simulink model "VCMGCM1962020b_v2"  (R2020b)
settings: Solver=FixedStepDiscrete  StartTime=0.0  StopTime=10.0  FixedStep=0.005  RelTol=1e-3  EnableMultiTasking=on
PreLoadFcn:
  | try, model_open; catch, disp('Error occurred while executing model pre-load callback: model_open.m'); disp('Please assure that the MATLAB working directory is set to the model directory before opening.'); end
InitFcn:
  | try, model_open; catch, end
undefined symbols (not defined in the file): Bridge, GCM, H, raptor_get_param_eval, raptor_get_safe_string, raptor_xcp_function
libraries: Blocks_lib x1165, Raptor_lib x665, simulink x62, VCM_lib x5
(part 8 of 23)

== system VCMGCM1962020b_v2/Fgnd/Actuators/CAN/Other/MPDM ==
  Data : Inport
  Ground : Ground
  Header : Blocks_lib/Header  width=Portrait  addtext=''
  MsgName : Subsystem
      mask help:
      | Example of how to set up a CAN message transmit.
      | 1. Copy this block into the main model.
      | 2. Disable/break library link.
      | 3. Underneath, set up CAN Tx Message block.
      | 4. For each field, connect a CANTxField block from the CAN block to the bus creator; adjust parameters as necessary.
      mask init:
      | [msgnam, msgbus] = CANBlockInit('Tx');
      mask Display: disp(['CAN Tx: Message\n' msgnam '\n' msgbus]);
  Act : Outport  VectorParamsAs1DForOutWhenUnconnected=off
  wires:
  Data/1 -> MsgName/1(Data)
  Ground/1 -> Act/1  "MPDM"

== system VCMGCM1962020b_v2/Fgnd/Actuators/CAN/Other/Power Steering Pump Inverter ==
  Data : Inport
  Ground : Ground
  Header : Blocks_lib/Header  width=Portrait  addtext=''
  MsgName : Subsystem
      mask help:
      | Example of how to set up a CAN message transmit.
      | 1. Copy this block into the main model.
      | 2. Disable/break library link.
      | 3. Underneath, set up CAN Tx Message block.
      | 4. For each field, connect a CANTxField block from the CAN block to the bus creator; adjust parameters as necessary.
      mask init:
      | [msgnam, msgbus] = CANBlockInit('Tx');
      mask Display: disp(['CAN Tx: Message\n' msgnam '\n' msgbus]);
  PSPInvtrHC1_Demands : Subsystem
      mask help:
      | Example of how to set up a CAN message transmit.
      | 1. Copy this block into the main model.
      | 2. Disable/break library link.
      | 3. Underneath, set up CAN Tx Message block.
      | 4. For each field, connect a CANTxField block from the CAN block to the bus creator; adjust parameters as necessary.
      mask init:
      | [msgnam, msgbus] = CANBlockInit('Tx');
      mask Display: disp(['CAN Tx: Message\n' msgnam '\n' msgbus]);
  PSPInvtrHC3_Battery_Demands : Subsystem
      mask help:
      | Example of how to set up a CAN message transmit.
      | 1. Copy this block into the main model.
      | 2. Disable/break library link.
      | 3. Underneath, set up CAN Tx Message block.
      | 4. For each field, connect a CANTxField block from the CAN block to the bus creator; adjust parameters as necessary.
      mask init:
      | [msgnam, msgbus] = CANBlockInit('Tx');
      mask Display: disp(['CAN Tx: Message\n' msgnam '\n' msgbus]);
  Act : Outport  VectorParamsAs1DForOutWhenUnconnected=off
  wires:
  Ground/1 -> Act/1  "PSPInvtr"
  Data/1 -> PSPInvtrHC1_Demands/1(Data), MsgName/1(Data), PSPInvtrHC3_Battery_Demands/1(Data)

== system VCMGCM1962020b_v2/Fgnd/Actuators/FMWS/MCU_130h/FMWS Enbl ==
  note: Vehicle is moving or ready to move
  note: Vehicle is moving while in neutral
  note: First two conditions being true would mean vehicle is in neutral
  In1 : Inport
  AND1 : Logic  Inputs=3  AllPortsSameDT=off  OutDataTypeStr=boolean
  Bus Selector : BusSelector  OutputSignals=Control.Mode.StartStop.RunMode [Bool],VirtualSensors.Driver.Drv [Bool],VirtualSensors.Driver.Rev [Bool],VirtualSensors.Spd.VehSpd [kph]
  Compare To Zero : simulink/Logic and Bit Operations/Compare To Zero  relop=>  OutDataTypeStr=boolean
  NOT : Logic  Operator=NOT  IconShape=distinctive  AllPortsSameDT=off  OutDataTypeStr=boolean
  NOT1 : Logic  Operator=NOT  IconShape=distinctive  AllPortsSameDT=off  OutDataTypeStr=boolean
  OR : Logic  Operator=OR  AllPortsSameDT=off  OutDataTypeStr=boolean
  raptor_measurement : Raptor_lib/Data Storage/raptor_measurement  paramName='FMWS_Enbl'  nameSource=Parameter  calDispType=Number  calEnum={'False', 'True'}  calGain=1.0  calOffset=0.0  calMax=inf  calMin=-inf  calFormat='-1'  calUnit='Enable condition met for FMWS'  calHelp='Enable condition met for FMWS'  calAccess=1  calFunction=raptor_xcp_function(gcb)  calVisible=on
      settings: SourceProductName=Raptor
  raptor_override : Raptor_lib/Data Storage/raptor_override  paramName='FMWS_Enbl'  nameSource=Parameter  measurement=None  calDispType=Number  calEnum={'False', 'True'}  calGain=1.0  calOffset=0.0  calMax=inf  calMin=-inf  calFormat='-1'  calUnit='Enable condition met for FMWS'  calHelp='Enable condition met for FMWS'  calAccess=1  calFunction="[raptor_xcp_function(gcb) '|'  'Override']"
      settings: SourceProductName=Raptor
  Out1 : Outport
  wires:
  NOT1/1 -> AND1/2
  Bus Selector/2 -> NOT/1  "<Drv [Bool]>"
  Bus Selector/3 -> NOT1/1  "<Rev [Bool]>"
  AND1/1 -> OR/2
  In1/1 -> Bus Selector/1
  Bus Selector/1 -> OR/1  "<RunMode [Bool]>"
  NOT/1 -> AND1/1
  Bus Selector/4 -> Compare To Zero/1  "<VehSpd [kph]>"
  Compare To Zero/1 -> AND1/3
  raptor_override/1 -> raptor_measurement/1, Out1/1
  OR/1 -> raptor_override/1

== system VCMGCM1962020b_v2/Fgnd/Actuators/FMWS/MCU_130h/MsgTx ==
  Data : Inport
  Enable : EnablePort
  Bus Selector : BusSelector  OutputSignals=Control.Other.Other.FMWS_StateGear [enum]
  CANTxField1 : Blocks_lib/CANTxField  custom=off  custom_nam='---'  custom_units='---'
  Header : Blocks_lib/Header  width=Landscape  addtext=''
  raptor_can_txmsg : Raptor_lib/CAN/raptor_can_txmsg  canDefinition=struct('dbcFile', 'FMWS.dbc','message', 'MCU_130h','comment', '','signals', {{'MCU_MotActuSpd','GearPos'}},'enabled', [ 0 1;],'scaled', [ 1 1;],'canBus', 'bus','messageID', [ 304;],'idMask', [ 536870911;],'payloadMask', [],'payloadValue', [],'period', [ 100;],'mailbox', '','queueSize', [ 1;],'label', [ 1;],'ver', [ 2;],'showID', [ 0;],'showRaw', [ 0;],'fill', [ 0;],'editID', [ 0;],'signalOrder', [ 3;],'signalAscDes', [ 1;])  canBus=bus  queueSize=1  payloadMask=[]  payloadValue=[]  period=100  showID=0  label=1  idMask=hex2dec('1FFFFFFF')  fill=0  id=304  showRaw=0  signalOrder=3  signalInfo={{struct('Name', 'MCU_MotActuSpd','Startbit', [ 0;],'SignalSize', [ 16;],'ByteOrder', 'LittleEndian','ValueType', 'UNSIGNED','Class', 'uint16','Signed', [ 0;],'Factor', [ 1;],'Offset', [ -32000;],'Min', [ -32000;],'Max', [ 32000;],'Units', 'Rpm','Comment', 'Motor actual speed','StartBit', [ 16;]),struct('Name', 'GearPos','Startbit', [ 0;],'SignalSize', [ 8;],'ByteOrder', 'LittleEndian','ValueType', 'UNSIGNED','Class', 'uint8','Signed', [ 0;],'Factor', [ 1;],'Offset', [ 0;],'Min', [ 0;],'Max', [ 0;],'Units', '','Comment', '','StartBit', [ 48;])}}
      settings: SourceProductName=Raptor
  wires:
  Data/1 -> Bus Selector/1
  CANTxField1/1 -> raptor_can_txmsg/1  "GearPos"
  Bus Selector/1 -> CANTxField1/1  "<FMWS_StateGear [enum]>"

== system VCMGCM1962020b_v2/Fgnd/Actuators/FMWS/MCU_131h/MsgTx ==
  Data : Inport
  Enable : EnablePort
  Bus Selector : BusSelector  OutputSignals=VirtualSensors.Spd.VehSpd [kph]
  CANTxField : Blocks_lib/CANTxField  custom=on  custom_nam=[nam '---']  custom_units='---'
  Header : Blocks_lib/Header  width=Landscape  addtext=''
  raptor_can_txmsg : Raptor_lib/CAN/raptor_can_txmsg  canDefinition=struct('dbcFile', 'FMWS.dbc','message', 'MCU_131h','comment', '','signals', {{'VehicleSpeed'}},'enabled', [ 1;],'scaled', [ 1;],'canBus', 'bus','messageID', [ 305;],'idMask', [ 536870911;],'payloadMask', [],'payloadValue', [],'period', [ 100;],'queueSize', [ 1;],'label', [ 1;],'ver', [ 2;],'showID', [ 0;],'showRaw', [ 0;],'showRawMsg', [ 0;],'useStartVals', [ 0;],'useSimFunc', [ 0;],'sim_func_name', '''''','fill', [ 0;],'editID', [ 0;],'signalOrder', [ 3;],'signalAscDes', [ 1;],'msgLength', [ 8;])  canBus=bus  queueSize=1  payloadMask=[]  payloadValue=[]  period=100  showID=0  label=1  idMask=hex2dec('1FFFFFFF')  fill=0  id=305  showRaw=0  signalOrder=3  signalInfo={{struct('Name', 'VehicleSpeed','Startbit', [ 0;],'SignalSize', [ 16;],'ByteOrder', 'LittleEndian','ValueType', 'SIGNED','Class', 'int16','Signed', [ 1;],'Factor', [ 0.0625;],'Offset', [ 0;],'Min', [ -100;],'Max', [ 100;],'Units', 'Km/hr','Comment', 'Speed','StartBit', [ 0;])}}
      settings: SourceProductName=Raptor
  wires:
  Bus Selector/1 -> CANTxField/1  "<VehSpd [kph]>"
  Data/1 -> Bus Selector/1
  CANTxField/1 -> raptor_can_txmsg/1  "VehicleSpeed"

== system VCMGCM1962020b_v2/Fgnd/Actuators/FMWS_J1939/CCVS/MsgTx ==
  Data : Inport
  Enable : EnablePort
  Bus Selector : BusSelector  OutputSignals=VirtualSensors.Spd.VehSpd [kph],VirtualSensors.Driver.Prk [Bool]
  CANTxField1 : Blocks_lib/CANTxField  custom=off  custom_nam='---'  custom_units='---'
  CANTxField2 : Blocks_lib/CANTxField  custom=off  custom_nam='---'  custom_units='---'
  Header : Blocks_lib/Header  width=Landscape  addtext=''
  raptor_can_txmsg : Raptor_lib/CAN/raptor_can_txmsg  canDefinition=struct('dbcFile', 'ECCO_EVAS.dbc','message', 'CCVS','comment', '','signals', {{'EngShutdownOverrideSwitch','EngTestModeSwitch','EngIdleDecrementSwitch','EngIdleIncrementSwitch','CruiseCtrlStates','PTOGovernorState','CruiseCtrlSetSpeed','CruiseCtrlAccelerateSwitch','CruiseCtrlResumeSwitch','CruiseCtrlCoastSwitch','CruiseCtrlSetSwitch','ClutchSwitch','BrakeSwitch','CruiseCtrlEnableSwitch','CruiseCtrlActive','WheelBasedVehicleSpeed','ParkBrakeReleaseInhibitRq','CruiseCtrlPauseSwitch','ParkingBrakeSwitch','TwoSpeedAxleSwitch'}},'enabled', [ 0 0 0 0 0 0 0 0 0 0 0 0 0 0 0 1 0 0 1 0;],'scaled', [ 1 1 1 1 1 1 1 1 1 1 1 1 1 1 1 1 1 1 1 1;],'canBus', 'bus','messageID', [ 419361024;],'idMask', [ 536870911;],'payloadMask', [],'payloadValue', [],'period', [ 100;],'mailbox', '','queueSize', [ 1;],'label', [ 1;],'ver', [ 2;],'showID', [ 0;],'showRaw', [ 0;],'fill', [ 0;],'editID', [ 0;],'signalOrder', [ 3;],'signalAscDes', [ 1;])  canBus=bus  queueSize=1  payloadMask=[]  payloadValue=[]  period=100  showID=0  label=1  idMask=hex2dec('1FFFFFFF')  fill=0  id=419361024  showRaw=0  signalOrder=3  signalInfo={{struct('Name', 'EngShutdownOverrideSwitch','Startbit', [ 0;],'SignalSize', [ 2;],'ByteOrder', 'LittleEndian','ValueType', 'UNSIGNED','Class', 'uint8','Signed', [ 0;],'Factor', [ 1;],'Offset', [ 0;],'Min', [ 0;],'Max', [ 3;],'Units', '','Comment', '','StartBit', [ 62;]),struct('Name', 'EngTestModeSwitch','Startbit', [ 0;],'SignalSize', [ 2;],'ByteOrder', 'LittleEndian','ValueType', 'UNSIGNED','Class', 'uint8','Signed', [ 0;],'Factor', [ 1;],'Offset', [ 0;],'Min', [ 0;],'Max', [ 3;],'Units', '','Comment', '','StartBit', [ 60;]),struct('Name', 'EngIdleDecrementSwitch','Startbit', [ 0;],'SignalSize', [ 2;],'ByteOrder', 'LittleEndian','ValueType', 'UNSIGNED','Class', 'uint8','Signed', [ 0;],'Factor', [ 1;],'Offset', [ 0;],'Min', [ 0;],'Max', [ 3;],'Units', '','Comment', '','StartBit', [ 58;]),struct('Name', 'EngIdleIncrementSwitch','Startbit', [ 0;],'SignalSize', [ 2;],'ByteOrder', 'LittleEndian','ValueType', 'UNSIGNED','Class', 'uint8','Signed', [ 0;],'Factor', [ 1;],'Offset', [ 0;],'Min', [ 0;],'Max', [ 3;],'Units', '','Comment', '','StartBit', [ 56;]),struct('Name', 'CruiseCtrlStates','Startbit', [ 0;],'SignalSize', [ 3;],'ByteOrder', 'LittleEndian','ValueType', 'UNSIGNED','Class', 'uint8','Signed', [ 0;],'Factor', [ 1;],'Offset', [ 0;],'Min', [ 0;],'Max', [ 7;],'Units', '','Comment', '','StartBit', [ 53;]),struct('Name', 'PTOGovernorState','Startbit', [ 0;],'SignalSize', [ 5;],'ByteOrder', 'LittleEndian','ValueType', 'UNSIGNED','Class', 'uint8','Signed', [ 0;],'Factor', [ 1;],'Offset', [ 0;],'Min', [ 0;],'Max', [ 31;],'Units', '','Comment', '','StartBit', [ 48;]),struct('Name', 'CruiseCtrlSetSpeed','Startbit', [ 0;],'SignalSize', [ 8;],'ByteOrder', 'LittleEndian','ValueType', 'UNSIGNED','Class', 'uint8','Signed', [ 0;],'Factor', [ 1;],'Offset', [ 0;],'Min', [ 0;],'Max', [ 250;],'Units', 'km/h','Comment', '','StartBit', [ 40;]),struct('Name', 'CruiseCtrlAccelerateSwitch','Startbit', [ 0;],'SignalSize', [ 2;],'ByteOrder', 'LittleEndian','ValueType', 'UNSIGNED','Class', 'uint8','Signed', [ 0;],'Factor', [ 1;],'Offset', [ 0;],'Min', [ 0;],'Max', [ 3;],'Units', '','Comment', '','StartBit', [ 38;]),struct('Name', 'CruiseCtrlResumeSwitch','Startbit', [ 0;],'SignalSize', [ 2;],'ByteOrder', 'LittleEndian','ValueType', 'UNSIGNED','Class', 'uint8','Signed', [ 0;],'Factor', [ 1;],'Offset', [ 0;],'Min', [ 0;],'Max', [ 3;],'Units', '','Comment', '','StartBit', [ 36;]),struct('Name', 'CruiseCtrlCoastSwitch','Startbit', [ 0;],'SignalSize', [ 2;],'ByteOrder', 'LittleEndian','ValueType', 'UNSIGNED','Class', 'uint8','Signed', [ 0;],'Factor', [ 1;],'Offset', [ 0;],'Min', [ 0;],'Max', [ 3;],'Units', '','Comment', '','StartBit', [ 34;]),struct('Name', 'CruiseCtrlSetSwitch','Startbit', [ 0;],'SignalSize', [ 2;],'ByteOrder', 'LittleEndian','ValueType', 'UNSIGNED','Class', 'uint8','Signed', [ 0;],'Factor', [ 1;],'Offset', [ 0;],'Min', [ 0;],'Max', [ 3;],'Units', '','Comment', '','StartBit', [ 32;]),struct('Name', 'ClutchSwitch','Startbit', [ 0;],'SignalSize', [ 2;],'ByteOrder', 'LittleEndian','ValueType', 'UNSIGNED','Class', 'uint8','Signed', [ 0;],'Factor', [ 1;],'Offset', [ 0;],'Min', [ 0;],'Max', [ 3;],'Units', '','Comment', '','StartBit', [ 30;]),struct('Name', 'BrakeSwitch','Startbit', [ 0;],'SignalSize', [ 2;],'ByteOrder', 'LittleEndian','ValueType', 'UNSIGNED','Class', 'uint8','Signed', [ 0;],'Factor', [ 1;],'Offset', [ 0;],'Min', [ 0;],'Max', [ 3;],'Units', '','Comment', '','StartBit', [ 28;]),struct('Name', 'CruiseCtrlEnableSwitch','Startbit', [ 0;],'SignalSize', [ 2;],'ByteOrder', 'LittleEndian','ValueType', 'UNSIGNED','Class', 'uint8','Signed', [ 0;],'Factor', [ 1;],'Offset', [ 0;],'Min', [ 0;],'Max', [ 3;],'Units', '','Comment', '','StartBit', [ 26;]),struct('Name', 'CruiseCtrlActive','Startbit', [ 0;],'SignalSize', [ 2;],'ByteOrder', 'LittleEndian','ValueType', 'UNSIGNED','Class', 'uint8','Signed', [ 0;],'Factor', [ 1;],'Offset', [ 0;],'Min', [ 0;],'Max', [ 3;],'Units', '','Comment', '','StartBit', [ 24;]),struct('Name', 'WheelBasedVehicleSpeed','Startbit', [ 0;],'SignalSize', [ 16;],'ByteOrder', 'LittleEndian','ValueType', 'UNSIGNED','Class', 'uint16','Signed', [ 0;],'Factor', [ 0.0039062;],'Offset', [ 0;],'Min', [ 0;],'Max', [ 250.996;],'Units', 'km/h','Comment', '','StartBit', [ 8;]),struct('Name', 'ParkBrakeReleaseInhibitRq','Startbit', [ 0;],'SignalSize', [ 2;],'ByteOrder', 'LittleEndian','ValueType', 'UNSIGNED','Class', 'uint8','Signed', [ 0;],'Factor', [ 1;],'Offset', [ 0;],'Min', [ 0;],'Max', [ 3;],'Units', '','Comment', '','StartBit', [ 6;]),struct('Name', 'CruiseCtrlPauseSwitch','Startbit', [ 0;],'SignalSize', [ 2;],'ByteOrder', 'LittleEndian','ValueType', 'UNSIGNED','Class', 'uint8','Signed', [ 0;],'Factor', [ 1;],'Offset', [ 0;],'Min', [ 0;],'Max', [ 3;],'Units', '','Comment', '','StartBit', [ 4;]),struct('Name', 'ParkingBrakeSwitch','Startbit', [ 0;],'SignalSize', [ 2;],'ByteOrder', 'LittleEndian','ValueType', 'UNSIGNED','Class', 'uint8','Signed', [ 0;],'Factor', [ 1;],'Offset', [ 0;],'Min', [ 0;],'Max', [ 3;],'Units', '','Comment', '','StartBit', [ 2;]),struct('Name', 'TwoSpeedAxleSwitch','Startbit', [ 0;],'SignalSize', [ 2;],'ByteOrder', 'LittleEndian','ValueType', 'UNSIGNED','Class', 'uint8','Signed', [ 0;],'Factor', [ 1;],'Offset', [ 0;],'Min', [ 0;],'Max', [ 3;],'Units', '','Comment', '','StartBit', [ 0;])}}
      settings: SourceProductName=Raptor
  wires:
  CANTxField1/1 -> raptor_can_txmsg/1  "WheelBasedVehicleSpeed"
  Data/1 -> Bus Selector/1
  Bus Selector/2 -> CANTxField2/1  "<Prk [Bool]>"
  CANTxField2/1 -> raptor_can_txmsg/2  "ParkingBrakeSwitch"
  Bus Selector/1 -> CANTxField1/1  "<VehSpd [kph]>"

== system VCMGCM1962020b_v2/Fgnd/Actuators/FMWS_J1939/ETC2/MsgTx ==
  Data : Inport
  Enable : EnablePort
  Bus Selector : BusSelector  OutputSignals=VirtualSensors.Spd.VehSpd [kph]
  CANTxField : Blocks_lib/CANTxField  custom=on  custom_nam=[nam '---']  custom_units='---'
  Header : Blocks_lib/Header  width=Landscape  addtext=''
  raptor_can_txmsg : Raptor_lib/CAN/raptor_can_txmsg  canDefinition=struct('dbcFile', 'ECCO_EVAS.dbc','message', 'ETC2','comment', '','signals', {{'TransCurrentRange','TransRequestedRange','TransCurrentGear','TransActualGearRatio','TransSelectedGear'}},'enabled', [ 0 0 1 0 0;],'scaled', [ 1 1 1 1 1;],'canBus', 'bus','messageID', [ 418383104;],'idMask', [ 536870911;],'payloadMask', [],'payloadValue', [],'period', [ 100;],'mailbox', '','queueSize', [ 1;],'label', [ 1;],'ver', [ 2;],'showID', [ 0;],'showRaw', [ 0;],'fill', [ 0;],'editID', [ 0;],'signalOrder', [ 3;],'signalAscDes', [ 1;])  canBus=bus  queueSize=1  payloadMask=[]  payloadValue=[]  period=100  showID=0  label=1  idMask=hex2dec('1FFFFFFF')  fill=0  id=418383104  showRaw=0  signalOrder=3  signalInfo={{struct('Name', 'TransCurrentRange','Startbit', [ 0;],'SignalSize', [ 16;],'ByteOrder', 'LittleEndian','ValueType', 'UNSIGNED','Class', 'uint16','Signed', [ 0;],'Factor', [ 1;],'Offset', [ 0;],'Min', [ 0;],'Max', [ 255;],'Units', 'per byte','Comment', '','StartBit', [ 48;]),struct('Name', 'TransRequestedRange','Startbit', [ 0;],'SignalSize', [ 16;],'ByteOrder', 'LittleEndian','ValueType', 'UNSIGNED','Class', 'uint16','Signed', [ 0;],'Factor', [ 1;],'Offset', [ 0;],'Min', [ 0;],'Max', [ 255;],'Units', 'per byte','Comment', '','StartBit', [ 32;]),struct('Name', 'TransCurrentGear','Startbit', [ 0;],'SignalSize', [ 8;],'ByteOrder', 'LittleEndian','ValueType', 'UNSIGNED','Class', 'uint8','Signed', [ 0;],'Factor', [ 1;],'Offset', [ -125;],'Min', [ -125;],'Max', [ 125;],'Units', '','Comment', '','StartBit', [ 24;]),struct('Name', 'TransActualGearRatio','Startbit', [ 0;],'SignalSize', [ 16;],'ByteOrder', 'LittleEndian','ValueType', 'UNSIGNED','Class', 'uint16','Signed', [ 0;],'Factor', [ 0.001;],'Offset', [ 0;],'Min', [ 0;],'Max', [ 64.255;],'Units', '','Comment', '','StartBit', [ 8;]),struct('Name', 'TransSelectedGear','Startbit', [ 0;],'SignalSize', [ 8;],'ByteOrder', 'LittleEndian','ValueType', 'UNSIGNED','Class', 'uint8','Signed', [ 0;],'Factor', [ 1;],'Offset', [ -125;],'Min', [ -125;],'Max', [ 125;],'Units', '','Comment', '','StartBit', [ 0;])}}
      settings: SourceProductName=Raptor
  wires:
  CANTxField/1 -> raptor_can_txmsg/1  "TransCurrentGear"
  Data/1 -> Bus Selector/1
  Bus Selector/1 -> CANTxField/1  "<VehSpd [kph]>"

== system VCMGCM1962020b_v2/Fgnd/Control/Drive Inverter/Motor Torque Request/Current//Torque Split ==
  Data : Inport
  TrqReq : Inport  Port=2
  Bus Creator : BusCreator  Inputs=3
  Bus Selector : BusSelector  OutputSignals=DrvTrqReqFinal [Nm]
  Constant : Constant  Value=double(1)
  Constant1 : Constant  Value=double(1)
  Constant2 : Constant  Value=double(1)
  Header : Blocks_lib/Header  width=Portrait  addtext=''
  Inverter Current Limits : Subsystem
  Product : Product
  Product1 : Product
  Product2 : Product
  Split : Outport  VectorParamsAs1DForOutWhenUnconnected=off
  wires:
  Product/1 -> Bus Creator/1  "DrvInvtrMCLSplit [A]"
  Bus Creator/1 -> Split/1  "Split"
  Product1/1 -> Bus Creator/2  "DrvInvtrGCLSplit [A]"
  Product2/1 -> Bus Creator/3  "DrvMtrTrqReqSplit [Nm]"
  Bus Selector/1 -> Product2/1  "<DrvTrqReqFinal [Nm]>"
  Constant/1 -> Product/2
  Constant1/1 -> Product1/2
  Constant2/1 -> Product2/2
  Inverter Current Limits/1(MCL) -> Product/1
  Data/1 -> Inverter Current Limits/1(Data)
  TrqReq/1 -> Bus Selector/1
  Inverter Current Limits/2(GCL) -> Product1/1

== system VCMGCM1962020b_v2/Fgnd/Control/Drive Inverter/Motor Torque Request/Driver Torque Request ==
  Data : Inport
  Bus Creator : BusCreator  Inputs=4
  Cruise Control : Subsystem  mask{group=[group ' | Cruise Control']}
  Driveability : Subsystem
  Header : Blocks_lib/Header  width=Portrait  addtext=''
  Pedal Torque Request : Subsystem
  Vehicle Speed Limiter : Subsystem
  TrqReq : Outport  VectorParamsAs1DForOutWhenUnconnected=off
  wires:
  Cruise Control/2(Nm) -> Driveability/2(DrvTrq)
  Cruise Control/1(CC) -> Bus Creator/3
  Vehicle Speed Limiter/1(kph) -> Bus Creator/2  "VehSpdLim [kph]"
  Data/1 -> Pedal Torque Request/1(Data), Driveability/1(Data), Cruise Control/1(Data), Vehicle Speed Limiter/1(Data)
  Driveability/1(Nm) -> Bus Creator/4  "DrvTrqReqFinal [Nm]"
  Pedal Torque Request/1(Nm) -> Vehicle Speed Limiter/2(DrvTrq), Bus Creator/1  "DrvTrqReqRaw [Nm]"
  Vehicle Speed Limiter/2(Nm) -> Cruise Control/2(DrvTrq)
  Bus Creator/1 -> TrqReq/1  "DrvTrqReq"

== system VCMGCM1962020b_v2/Fgnd/Control/Drive Inverter/Motor Torque Request/Inverter//Motor Limit & Request ==
  Data : Inport
  EnblReq : Inport  Port=2
  Split : Inport  Port=3
  BusCreator : BusCreator  Inputs=3
  Header : Blocks_lib/Header  width=Portrait  addtext=''
  Inverter Current Limit : Subsystem
  Motor Torque Limit : Subsystem
  Motor Torque Request : Subsystem
  raptor_measurement : Raptor_lib/Data Storage/raptor_measurement  paramName=[mtrnam 'TrqReq']  nameSource=Parameter  calDispType=Number  calEnum={'Disabled', 'Enabled'}  calGain=1  calOffset=0  calMax=inf  calMin=-inf  calFormat=''  calUnit='Nm'  calHelp='Motor torque limit'  calAccess=1  calFunction=group  calVisible=on
      settings: SourceProductName=Raptor
  InvtrMtr : Outport  VectorParamsAs1DForOutWhenUnconnected=off
  wires:
  Motor Torque Limit/1(Nm) -> Motor Torque Request/4(TrqLim), BusCreator/2  "DrvMtrTrqLim [Nm]"
  Inverter Current Limit/1(InvtrCurLim) -> Motor Torque Limit/3(InvtrCurLim), BusCreator/1
  BusCreator/1 -> InvtrMtr/1  "DrvInvtr"
  Data/1 -> Motor Torque Request/1(Data), Motor Torque Limit/1(Data)
  Motor Torque Request/1(Nm) -> raptor_measurement/1, BusCreator/3  "DrvMtrTrqReq [Nm]"
  EnblReq/1 -> Motor Torque Request/2(EnblReq), Motor Torque Limit/2(EnblReq)
  Split/1 -> Motor Torque Request/3("Split "), Inverter Current Limit/1(Split)

== system VCMGCM1962020b_v2/Fgnd/Control/Modes/PRND Mode/AllowShiftFromPark ==
  Data : Inport
  Bus Selector : BusSelector  OutputSignals=VirtualSensors.Driver.BrkSw [Bool],VirtualSensors.Chgr.ChgPlugState [enum]
  CmprTo : Blocks_lib/CmprTo  op===  val='Disconnected'  enum=EnumLst.ChgPlugState
  Header : Blocks_lib/Header  width=Portrait  addtext=''
  Logical Operator : Logic  AllPortsSameDT=off  OutDataTypeStr=boolean
  Bool : Outport  VectorParamsAs1DForOutWhenUnconnected=off
  wires:
  Data/1 -> Bus Selector/1
  Bus Selector/1 -> Logical Operator/1  "<BrkSw [Bool]>"
  CmprTo/1 -> Logical Operator/2
  Bus Selector/2 -> CmprTo/1  "<ChgPlugState [enum]>"
  Logical Operator/1 -> Bool/1

== system VCMGCM1962020b_v2/Fgnd/Control/Modes/PRND Mode/PRND ==
  note: Note: a Park request has the highest priority, followed by Neutral, Drive, and then Reverse.
  Data : Inport
  Bus Selector : BusSelector  OutputSignals=VirtualSensors.Driver.Prk [Bool]
  Bus Selector1 : BusSelector  OutputSignals=VirtualSensors.Driver.Prk [Bool],VirtualSensors.Driver.Rev [Bool],VirtualSensors.Driver.Ntrl [Bool],VirtualSensors.Driver.Drv [Bool]
  Bus Selector2 : BusSelector  OutputSignals=VirtualSensors.Driver.Prk [Bool],VirtualSensors.Driver.Ntrl [Bool]
  Bus Selector3 : BusSelector  OutputSignals=VirtualSensors.Driver.Prk [Bool],VirtualSensors.Driver.Ntrl [Bool],VirtualSensors.Driver.Drv [Bool]
  Header : Blocks_lib/Header  width=Portrait  addtext=''
  Logical Operator : Logic  Inputs=4  OutDataTypeStr=boolean
  Logical Operator1 : Logic  OutDataTypeStr=boolean
  Logical Operator2 : Logic  Inputs=3  OutDataTypeStr=boolean
  Logical Operator{3..8} (6 alike) : Logic  Operator=NOT  Inputs=1  OutDataTypeStr=boolean
  P : Outport  VectorParamsAs1DForOutWhenUnconnected=off
  R : Outport  Port=2  VectorParamsAs1DForOutWhenUnconnected=off
  N : Outport  Port=3  VectorParamsAs1DForOutWhenUnconnected=off
  D : Outport  Port=4  VectorParamsAs1DForOutWhenUnconnected=off
  wires:
  Bus Selector/1 -> P/1  "<Prk [Bool]>"
  Bus Selector2/2 -> Logical Operator1/2  "<Ntrl [Bool]>"
  Bus Selector1/1 -> Logical Operator3/1  "<Prk [Bool]>"
  Bus Selector1/2 -> Logical Operator/2  "<Rev [Bool]>"
  Bus Selector1/3 -> Logical Operator4/1  "<Ntrl [Bool]>"
  Bus Selector1/4 -> Logical Operator5/1  "<Drv [Bool]>"
  Logical Operator4/1 -> Logical Operator/3
  Logical Operator5/1 -> Logical Operator/4
  Logical Operator2/1 -> D/1
  Logical Operator3/1 -> Logical Operator/1
  Bus Selector3/1 -> Logical Operator7/1  "<Prk [Bool]>"
  Bus Selector3/2 -> Logical Operator8/1  "<Ntrl [Bool]>"
  Bus Selector3/3 -> Logical Operator2/3  "<Drv [Bool]>"
  Logical Operator7/1 -> Logical Operator2/1
  Logical Operator8/1 -> Logical Operator2/2
  Logical Operator/1 -> R/1
  Data/1 -> Bus Selector/1, Bus Selector1/1, Bus Selector3/1, Bus Selector2/1
  Bus Selector2/1 -> Logical Operator6/1  "<Prk [Bool]>"
  Logical Operator6/1 -> Logical Operator1/1
  Logical Operator1/1 -> N/1

== system VCMGCM1962020b_v2/Fgnd/Control/Modes/Startup & Shutdown/Battery Charge Required ==
  Data : Inport
  Bus Selector : BusSelector  OutputSignals=VirtualSensors.Batt.BattChgComplete [Bool]
  Bus Selector1 : BusSelector  OutputSignals=Sensors.Sensors.Volt.DRVPVolt.DRVPVolt [V]
  Header : Blocks_lib/Header  width=Portrait  addtext=''
  Logical Operator : Logic  Operator=NOT  Inputs=1  AllPortsSameDT=off  OutDataTypeStr=boolean
  Relational Operator : RelationalOperator  Operator=<=  OutDataTypeStr=boolean  RndMeth=Simplest
  raptor_adjustment : Raptor_lib/Data Storage/raptor_adjustment  paramName='LVBattChgReqdThr'  nameSource=Parameter  initValue=0  dataType=double  storage=Calibration  calDispType=Number  calEnum={'Disabled', 'Enabled'}  calGain=1  calOffset=0  calMax=inf  calMin=-inf  calFormat=''  calUnit='V'  calHelp='Low-voltage battery charge required threshold (on DRVP voltage)'  calAccess=1  calFunction=group  calDispHeaders=off  calColHeaders={'Col1' 'Col2' 'Col3'}  calRowHeaders={'Row1' 'Row2' 'Row3'}
      settings: SourceProductName=Raptor
  raptor_measurement : Raptor_lib/Data Storage/raptor_measurement  paramName='HVBattChgReqd'  nameSource=Parameter  calDispType=Number  calEnum={'Disabled', 'Enabled'}  calGain=1  calOffset=0  calMax=inf  calMin=-inf  calFormat=''  calUnit='Bool'  calHelp='High-voltage battery charge required'  calAccess=1  calFunction=group  calVisible=on
      settings: SourceProductName=Raptor
  raptor_measurement1 : Raptor_lib/Data Storage/raptor_measurement  paramName='LVBattChgReqd'  nameSource=Parameter  calDispType=Number  calEnum={'Disabled', 'Enabled'}  calGain=1  calOffset=0  calMax=inf  calMin=-inf  calFormat=''  calUnit='Bool'  calHelp='Low-voltage battery charge required'  calAccess=1  calFunction=group  calVisible=on
      settings: SourceProductName=Raptor
  HV : Outport  VectorParamsAs1DForOutWhenUnconnected=off
  LV : Outport  Port=2  VectorParamsAs1DForOutWhenUnconnected=off
  wires:
  Data/1 -> Bus Selector1/1, Bus Selector/1
  Logical Operator/1 -> HV/1, raptor_measurement/1
  Bus Selector/1 -> Logical Operator/1  "<BattChgComplete [Bool]>"
  Bus Selector1/1 -> Relational Operator/1  "<DRVPVolt [V]>"
  Relational Operator/1 -> LV/1, raptor_measurement1/1
  raptor_adjustment/1 -> Relational Operator/2

== system VCMGCM1962020b_v2/Fgnd/Control/Modes/Startup & Shutdown/HV No Detect ==
  Data : Inport
  Bus Selector : BusSelector  OutputSignals=VirtualSensors.PDU.HVBusVolt [V]
  Header : Blocks_lib/Header  width=Portrait  addtext=''
  Relational Operator : RelationalOperator  Operator=<=  OutDataTypeStr=boolean  RndMeth=Nearest
  raptor_adjustment : Raptor_lib/Data Storage/raptor_adjustment  paramName='HVNoDetectThr'  nameSource=Parameter  initValue=0  dataType=double  storage=Calibration  calDispType=Number  calEnum={'Disabled', 'Enabled'}  calGain=1  calOffset=0  calMax=inf  calMin=-inf  calFormat=''  calUnit='V'  calHelp='High voltage not detected threshold (post battery contactors)'  calAccess=1  calFunction=group  calDispHeaders=off  calColHeaders={'Col1' 'Col2' 'Col3'}  calRowHeaders={'Row1' 'Row2' 'Row3'}
      settings: SourceProductName=Raptor
  raptor_measurement : Raptor_lib/Data Storage/raptor_measurement  paramName='HVNoDetect'  nameSource=Parameter  calDispType=Number  calEnum={'Disabled', 'Enabled'}  calGain=1  calOffset=0  calMax=inf  calMin=-inf  calFormat=''  calUnit='Bool'  calHelp='High voltage not detected (post battery contactors)'  calAccess=1  calFunction=group  calVisible=on
      settings: SourceProductName=Raptor
  Bool : Outport  VectorParamsAs1DForOutWhenUnconnected=off
  wires:
  Data/1 -> Bus Selector/1
  Bus Selector/1 -> Relational Operator/1  "<HVBusVolt [V]>"
  raptor_adjustment/1 -> Relational Operator/2
  Relational Operator/1 -> raptor_measurement/1, Bool/1

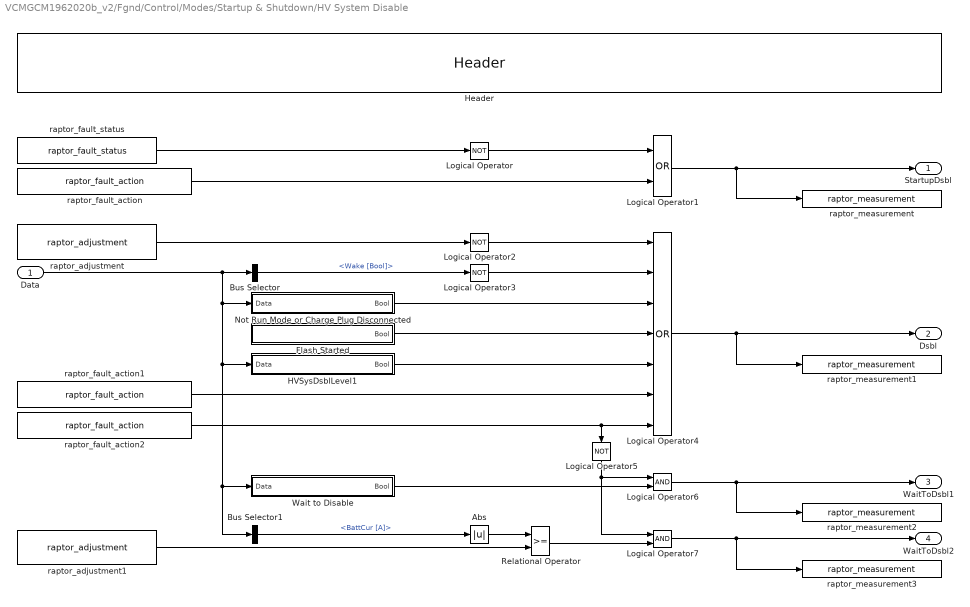
== system VCMGCM1962020b_v2/Fgnd/Control/Modes/Startup & Shutdown/HV System Disable ==
  Data : Inport
  Abs : Abs
  Bus Selector : BusSelector  OutputSignals=Sensors.Sensors.Volt.Wake [Bool]
  Bus Selector1 : BusSelector  OutputSignals=VirtualSensors.Batt.BattCur [A]
  Flash Started : Subsystem
  HVSysDsblLevel1 : Subsystem
  Header : Blocks_lib/Header  width=Portrait  addtext=''
  Logical Operator : Logic  Operator=NOT  Inputs=1  AllPortsSameDT=off  OutDataTypeStr=boolean
  Logical Operator1 : Logic  Operator=OR  AllPortsSameDT=off  OutDataTypeStr=boolean
  Logical Operator2 : Logic  Operator=NOT  Inputs=1  OutDataTypeStr=boolean
  Logical Operator3 : Logic  Operator=NOT  Inputs=1  OutDataTypeStr=boolean
  Logical Operator4 : Logic  Operator=OR  Inputs=7  OutDataTypeStr=boolean
  Logical Operator5 : Logic  Operator=NOT  Inputs=1  OutDataTypeStr=boolean
  Logical Operator6 : Logic  OutDataTypeStr=boolean
  Logical Operator7 : Logic  OutDataTypeStr=boolean
  Not Run Mode or Charge Plug Disconnected : Subsystem
  Relational Operator : RelationalOperator  OutDataTypeStr=boolean  RndMeth=Nearest
  Wait to Disable : Subsystem
  raptor_adjustment : Raptor_lib/Data Storage/raptor_adjustment  paramName='HVSysEnbl'  nameSource=Parameter  initValue=0  dataType=boolean  storage=Calibration  calDispType=Number  calEnum={'False', 'True'}  calGain=1  calOffset=0  calMax=inf  calMin=-inf  calFormat=''  calUnit='Bool'  calHelp='High-voltage system enable'  calAccess=1  calFunction=group  calDispHeaders=off  calColHeaders={'Col1' 'Col2' 'Col3'}  calRowHeaders={'Row1' 'Row2' 'Row3'}
      settings: SourceProductName=Raptor
  raptor_adjustment1 : Raptor_lib/Data Storage/raptor_adjustment  paramName='HVSysDsblBattCurMx'  nameSource=Parameter  initValue=0  dataType=double  storage=Calibration  calDispType=Number  calEnum={'False', 'True'}  calGain=1  calOffset=0.0  calMax=inf  calMin=-inf  calFormat=''  calUnit='A'  calHelp='High-voltage system disable battery current maximum'  calAccess=1  calFunction=group  calDispHeaders=off  calColHeaders={'Col1' 'Col2' 'Col3'}  calRowHeaders={'Row1' 'Row2' 'Row3'}
      settings: SourceProductName=Raptor
  raptor_fault_action : Raptor_lib/Faults/raptor_fault_action  actionName='HVSysStartupDsbl'  calVisible=off  calAccess=1  calFunction='System | FaultManager | FaultAction'
      settings: SourceProductName=Raptor
  raptor_fault_action1 : Raptor_lib/Faults/raptor_fault_action  actionName='HVSysDsblLevel2'  calVisible=off  calAccess=1  calFunction='System | FaultManager | FaultAction'
      settings: SourceProductName=Raptor
  raptor_fault_action2 : Raptor_lib/Faults/raptor_fault_action  actionName='HVSysDsblLevel3'  calVisible=off  calAccess=1  calFunction='System | FaultManager | FaultAction'
      settings: SourceProductName=Raptor
  raptor_fault_status : Raptor_lib/Faults/raptor_fault_status  faultSource=Parameter  faultName='HVILXChk'  notOccurred=off  suspected=off  active=off  occurred=off  failedThisDC=off  testCmpltThisDC=on  failing=off  pending=off  confirmed=off  mil=off  permanent=off  ready=off  prevConfirmed=off  failedSinceClear=off  failedLastDC=off  prevMil=off
      settings: SourceProductName=Raptor
  raptor_measurement : Raptor_lib/Data Storage/raptor_measurement  paramName='HVSysStartupDsbl'  nameSource=Parameter  calDispType=Number  calEnum={'Disabled', 'Enabled'}  calGain=1  calOffset=0  calMax=inf  calMin=-inf  calFormat=''  calUnit='Bool'  calHelp='High-voltage system startup disable'  calAccess=1  calFunction=group  calVisible=on
      settings: SourceProductName=Raptor
  raptor_measurement1 : Raptor_lib/Data Storage/raptor_measurement  paramName='HVSysDsbl'  nameSource=Parameter  calDispType=Number  calEnum={'Disabled', 'Enabled'}  calGain=1  calOffset=0  calMax=inf  calMin=-inf  calFormat=''  calUnit='Bool'  calHelp='High-voltage system disable'  calAccess=1  calFunction=group  calVisible=on
      settings: SourceProductName=Raptor
  raptor_measurement2 : Raptor_lib/Data Storage/raptor_measurement  paramName='HVSysWaitToDsbl1'  nameSource=Parameter  calDispType=Number  calEnum={'Disabled', 'Enabled'}  calGain=1  calOffset=0  calMax=inf  calMin=-inf  calFormat=''  calUnit='Bool'  calHelp='High-voltage system wait to disable (due to vehicle state)'  calAccess=1  calFunction=group  calVisible=on
      settings: SourceProductName=Raptor
  raptor_measurement3 : Raptor_lib/Data Storage/raptor_measurement  paramName='HVSysWaitToDsbl2'  nameSource=Parameter  calDispType=Number  calEnum={'Disabled', 'Enabled'}  calGain=1  calOffset=0  calMax=inf  calMin=-inf  calFormat=''  calUnit='Bool'  calHelp='High-voltage system wait to disable (due to battery current)'  calAccess=1  calFunction=group  calVisible=on
      settings: SourceProductName=Raptor
  StartupDsbl : Outport  VectorParamsAs1DForOutWhenUnconnected=off
  Dsbl : Outport  Port=2  VectorParamsAs1DForOutWhenUnconnected=off
  WaitToDsbl1 : Outport  Port=3  VectorParamsAs1DForOutWhenUnconnected=off
  WaitToDsbl2 : Outport  Port=4  VectorParamsAs1DForOutWhenUnconnected=off
  wires:
  Logical Operator6/1 -> raptor_measurement2/1, WaitToDsbl1/1
  Logical Operator7/1 -> raptor_measurement3/1, WaitToDsbl2/1
  Not Run Mode or Charge Plug Disconnected/1(Bool) -> Logical Operator4/3
  raptor_fault_action1/1 -> Logical Operator4/6
  HVSysDsblLevel1/1(Bool) -> Logical Operator4/5
  Flash Started/1(Bool) -> Logical Operator4/4
  Data/1 -> Wait to Disable/1(Data), Bus Selector1/1, HVSysDsblLevel1/1(Data), Not Run Mode or Charge Plug Disconnected/1(Data), Bus Selector/1
  raptor_fault_action2/1 -> Logical Operator5/1, Logical Operator4/7
  Bus Selector/1 -> Logical Operator3/1  "<Wake [Bool]>"
  Bus Selector1/1 -> Abs/1  "<BattCur [A]>"
  raptor_adjustment/1 -> Logical Operator2/1
  Logical Operator3/1 -> Logical Operator4/2
  Logical Operator2/1 -> Logical Operator4/1
  Relational Operator/1 -> Logical Operator7/2
  Wait to Disable/1(Bool) -> Logical Operator6/2
  Abs/1 -> Relational Operator/1
  raptor_adjustment1/1 -> Relational Operator/2
  Logical Operator5/1 -> Logical Operator6/1, Logical Operator7/1
  Logical Operator4/1 -> raptor_measurement1/1, Dsbl/1
  Logical Operator1/1 -> raptor_measurement/1, StartupDsbl/1
  raptor_fault_action/1 -> Logical Operator1/2
  Logical Operator/1 -> Logical Operator1/1
  raptor_fault_status/1 -> Logical Operator/1

== system VCMGCM1962020b_v2/Fgnd/Control/Modes/Startup & Shutdown/On//Off ==
  Data : Inport
  Bus Selector : BusSelector  OutputSignals=Sensors.Sensors.Volt.Wake [Bool]
  Bus Selector1 : BusSelector  OutputSignals=Sensors.Sensors.Volt.Wake [Bool]
  Header : Blocks_lib/Header  width=Portrait  addtext=''
  Logical Operator : Logic  OutDataTypeStr=boolean
  Logical Operator1 : Logic  Operator=NOT  Inputs=1  OutDataTypeStr=boolean
  Logical Operator3 : Logic  Operator=NOT  Inputs=1  OutDataTypeStr=boolean
  raptor_fault_action : Raptor_lib/Faults/raptor_fault_action  actionName='KeepVCMOn'  calVisible=off  calAccess=1  calFunction='System | FaultManager | FaultAction'
      settings: SourceProductName=Raptor
  On : Outport  VectorParamsAs1DForOutWhenUnconnected=off
  Off : Outport  Port=2  VectorParamsAs1DForOutWhenUnconnected=off
  wires:
  Bus Selector/1 -> On/1  "<Wake [Bool]>"
  Logical Operator/1 -> Off/1
  Logical Operator1/1 -> Logical Operator/1
  Bus Selector1/1 -> Logical Operator1/1  "<Wake [Bool]>"
  Logical Operator3/1 -> Logical Operator/2
  raptor_fault_action/1 -> Logical Operator3/1
  Data/1 -> Bus Selector/1, Bus Selector1/1

== system VCMGCM1962020b_v2/Fgnd/Control/Other/A//C Compressor/Speed Request ==
  Data : Inport
  Reset : EnablePort  StatesWhenEnabling=reset
  Add : Sum
  Bus Selector : BusSelector  OutputSignals=VirtualSensors.Other.AmbientAirTemp [degC],VirtualSensors.Other.ACPress [kPa]
  Header : Blocks_lib/Header  width=Portrait  addtext=''
  PIDCtrl : Blocks_lib/PIDCtrl  nam='ACCSpdCtrl'  inunits='kPa'  units='rpm'  group='Control | AC Compressor'  samptime=samptime
  RateLim : Blocks_lib/RateLim  samptime=samptime
  raptor_adjustment : Raptor_lib/Data Storage/raptor_adjustment  paramName='ACCSpdReqRateLim'  nameSource=Parameter  initValue=zeros(1,2)  dataType=double  storage=Calibration  calDispType=Number  calEnum={'Disabled', 'Enabled'}  calGain=1  calOffset=0  calMax=inf  calMin=-inf  calFormat=''  calUnit='rpm/s'  calHelp='A/C compressor speed request rate limit'  calAccess=1  calFunction='Control | AC Compressor'  calDispHeaders=off  calColHeaders={'Col1' 'Col2' 'Col3'}  calRowHeaders={'Row1' 'Row2' 'Row3'}
      settings: SourceProductName=Raptor
  raptor_table_1d : Raptor_lib/Table Lookup/raptor_table_1d  dataName='ACPressSetptTbl'  initValue=zeros(1,11)  dataType=double  storage=Calibration  initValueX=[1:11]  dataTypeXY=double  storageXY=Calibration  calVisible=on  showTable=on  calGain=1.0  calOffset=0.0  calMax=Inf  calMin=-Inf  calFormat=''  calUnit='kPa'  calHelp='A/C pressure set point'  showBreakpoint=on  dataNameX='AmbientAirTemp11IdxArr'  calGainX=1.0  calOffsetX=0.0  calMaxX=Inf  calMinX=-Inf  calFormatX=''  calUnitX='degC'  calHelpX='Index array'  calAccess=1  calFunction='Control | AC Compressor'  measureEnable=on  mName='ACPressSetpt'
      settings: SourceProductName=Raptor
  raptor_table_1d1 : Raptor_lib/Table Lookup/raptor_table_1d  dataName='ACCSpdCtrlFeedFwdTbl'  initValue=zeros(1,11)  dataType=double  storage=Calibration  initValueX=[1:11]  dataTypeXY=double  storageXY=Calibration  calVisible=on  showTable=on  calGain=1.0  calOffset=0.0  calMax=Inf  calMin=-Inf  calFormat=''  calUnit='rpm'  calHelp='A/C speed control feedforward table'  showBreakpoint=on  dataNameX='ACPressSetpt11IdxArr'  calGainX=1.0  calOffsetX=0.0  calMaxX=Inf  calMinX=-Inf  calFormatX=''  calUnitX='kPa'  calHelpX='Index array'  calAccess=1  calFunction='Control | AC Compressor'  measureEnable=on  mName='ACCSpdCtrlFeedFwd'
      settings: SourceProductName=Raptor
  rpm : Outport  OutputWhenDisabled=reset  InitialOutput=0  VectorParamsAs1DForOutWhenUnconnected=off
  wires:
  Data/1 -> Bus Selector/1
  Bus Selector/1 -> raptor_table_1d/1  "<AmbientAirTemp [degC]>"
  Bus Selector/2 -> PIDCtrl/2  "<ACPress [kPa]>"
  RateLim/1 -> rpm/1
  raptor_adjustment/1 -> RateLim/2
  raptor_table_1d1/1 -> Add/1
  PIDCtrl/1 -> Add/2
  Add/1 -> RateLim/1
  raptor_table_1d/1 -> raptor_table_1d1/1, PIDCtrl/1

== system VCMGCM1962020b_v2/Fgnd/Control/Other/Cooling Pumps/Pump 1 Speed Request ==
  Data : Inport
  Bus Selector : BusSelector  OutputSignals=VirtualSensors.Batt.BattCellTempMx [degC]
  Fcn : Fcn  Commented=on  Expr=u(2) + (u(3) - u(2)) * u(1) / 100
  Header : Blocks_lib/Header  width=Portrait  addtext=''
  LinPct(w/Hyst) : Blocks_lib/LinPct(w//Hyst)  nam='CoolPump1SpdReq'  innam='BattTemp'  inunits='degC'  group='Control | Cooling Loop'
  Meas&Ovrd1 : Blocks_lib/Meas&Ovrd  nam='CoolPmp1'  name_source=Parameter  view_as=Number  enum_struct={}  gain=1  min=-inf  max=inf  precision=''  units='%'  help='Coolant pump 1 override'  group='Group'
  Mux2 : Mux  Commented=on  Inputs=3
  TimeHyst : Blocks_lib/TimeHyst  nam='CoolPump1'  group='Control | Cooling Loop'  samptime=samptime
  raptor_adjustment : Raptor_lib/Data Storage/raptor_adjustment  Commented=on  paramName='CoolPump1SpdReqMn'  nameSource=Parameter  initValue=0  dataType=double  storage=Calibration  calDispType=Number  calEnum={'False', 'True'}  calGain=1.0  calOffset=0.0  calMax=inf  calMin=-inf  calFormat=''  calUnit='rpm'  calHelp='Cooling pump speed request minimum'  calAccess=1  calFunction='Control | Cooling Loop'  calDispHeaders=off  calColHeaders={'Col1' 'Col2' 'Col3'}  calRowHeaders={'Row1' 'Row2' 'Row3'}
      settings: SourceProductName=Raptor
  raptor_adjustment1 : Raptor_lib/Data Storage/raptor_adjustment  Commented=on  paramName='CoolPump1SpdReqMx'  nameSource=Parameter  initValue=0  dataType=double  storage=Calibration  calDispType=Number  calEnum={'False', 'True'}  calGain=1.0  calOffset=0.0  calMax=inf  calMin=-inf  calFormat=''  calUnit='rpm'  calHelp='Cooling pump speed request maximum'  calAccess=1  calFunction='Control | Cooling Loop'  calDispHeaders=off  calColHeaders={'Col1' 'Col2' 'Col3'}  calRowHeaders={'Row1' 'Row2' 'Row3'}
      settings: SourceProductName=Raptor
  Bool : Outport  VectorParamsAs1DForOutWhenUnconnected=off
  % : Outport  Port=2  VectorParamsAs1DForOutWhenUnconnected=off
  wires:
  Data/1 -> Bus Selector/1
  raptor_adjustment/1 -> Mux2/2
  Mux2/1 -> Fcn/1
  raptor_adjustment1/1 -> Mux2/3
  TimeHyst/1 -> Bool/1
  LinPct(w/Hyst)/2 -> Meas&Ovrd1/1, Mux2/1
  LinPct(w/Hyst)/1 -> TimeHyst/1
  Bus Selector/1 -> LinPct(w/Hyst)/1  "<BattCellTempMx [degC]>"
  Meas&Ovrd1/1 -> %/1

== system VCMGCM1962020b_v2/Fgnd/Control/Other/Cooling Pumps/Pump 2 Speed Request ==
  Data : Inport
  Bus Selector : BusSelector  OutputSignals=VirtualSensors.Chgr.OnBoard.OnBoardChgrOverTemp [Bool],VirtualSensors.Chgr.OnBoard.OnBoardChgrTemp [degC],VirtualSensors.DCDC.DCDCTemp [degC],VirtualSensors.DrvInvtr.DrvInvtrTemp [degC]
  Bus Selector1 : BusSelector  OutputSignals=VirtualSensors.DrvInvtr.DrvMtrTemp [degC]
  Fcn : Fcn  Commented=on  Expr=u(2) + (u(3) - u(2)) * u(1) / 100
  Header : Blocks_lib/Header  width=Portrait  addtext=''
  LinPct(w/Hyst) : Blocks_lib/LinPct(w//Hyst)  nam='CoolPump2SpdReq'  innam='PwrElecTemp'  inunits='degC'  group='Control | Cooling Loop'
  LinPct(w/Hyst)1 : Blocks_lib/LinPct(w//Hyst)  nam='CoolPump2SpdReq'  innam='MtrTemp'  inunits='degC'  group='Control | Cooling Loop'
  Logical Operator : Logic  Operator=OR  Inputs=1  AllPortsSameDT=off  OutDataTypeStr=boolean
  Meas&Ovrd : Blocks_lib/Meas&Ovrd  nam='CoolPmp2'  name_source=Parameter  view_as=Number  enum_struct={}  gain=1  min=-inf  max=inf  precision=''  units='%'  help='Coolant pump 2 override'  group='Group'
  MinMax : MinMax  Function=max  Inputs=3
  MinMax1 : MinMax  Function=max
  Mux : Mux  Inputs=2
  Mux1 : Mux  Inputs=2
  Mux2 : Mux  Commented=on  Inputs=3
  OR : Logic  Operator=OR  AllPortsSameDT=off  OutDataTypeStr=boolean
  TimeHyst : Blocks_lib/TimeHyst  nam='CoolPump2'  group='Control | Cooling Loop'  samptime=samptime
  raptor_adjustment : Raptor_lib/Data Storage/raptor_adjustment  Commented=on  paramName='CoolPump2SpdReqMn'  nameSource=Parameter  initValue=0  dataType=double  storage=Calibration  calDispType=Number  calEnum={'False', 'True'}  calGain=1.0  calOffset=0.0  calMax=inf  calMin=-inf  calFormat=''  calUnit='rpm'  calHelp='Cooling pump speed request minimum'  calAccess=1  calFunction='Control | Cooling Loop'  calDispHeaders=off  calColHeaders={'Col1' 'Col2' 'Col3'}  calRowHeaders={'Row1' 'Row2' 'Row3'}
      settings: SourceProductName=Raptor
  raptor_adjustment1 : Raptor_lib/Data Storage/raptor_adjustment  Commented=on  paramName='CoolPump2SpdReqMx'  nameSource=Parameter  initValue=0  dataType=double  storage=Calibration  calDispType=Number  calEnum={'False', 'True'}  calGain=1.0  calOffset=0.0  calMax=inf  calMin=-inf  calFormat=''  calUnit='rpm'  calHelp='Cooling pump speed request maximum'  calAccess=1  calFunction='Control | Cooling Loop'  calDispHeaders=off  calColHeaders={'Col1' 'Col2' 'Col3'}  calRowHeaders={'Row1' 'Row2' 'Row3'}
      settings: SourceProductName=Raptor
  Bool : Outport  VectorParamsAs1DForOutWhenUnconnected=off
  % : Outport  Port=2  VectorParamsAs1DForOutWhenUnconnected=off
  wires:
  Bus Selector1/1 -> LinPct(w/Hyst)1/1  "<DrvMtrTemp [degC]>"
  LinPct(w/Hyst)/2 -> Mux1/2
  LinPct(w/Hyst)1/2 -> Mux1/1
  Bus Selector/2 -> MinMax/1  "<OnBoardChgrTemp [degC]>"
  Bus Selector/4 -> MinMax/3  "<DrvInvtrTemp [degC]>"
  Bus Selector/3 -> MinMax/2  "<DCDCTemp [degC]>"
  MinMax/1 -> LinPct(w/Hyst)/1
  raptor_adjustment1/1 -> Mux2/3
  Mux2/1 -> Fcn/1
  raptor_adjustment/1 -> Mux2/2
  Data/1 -> Bus Selector/1, Bus Selector1/1
  Logical Operator/1 -> TimeHyst/1
  LinPct(w/Hyst)1/1 -> Mux/2
  Mux/1 -> Logical Operator/1
  Mux1/1 -> MinMax1/1
  MinMax1/1 -> Meas&Ovrd/1, Mux2/1
  Meas&Ovrd/1 -> %/1
  LinPct(w/Hyst)/1 -> Mux/1
  Bus Selector/1 -> OR/1  "<OnBoardChgrOverTemp [Bool]>"
  TimeHyst/1 -> OR/2
  OR/1 -> Bool/1

== system VCMGCM1962020b_v2/Fgnd/Control/Other/Other/Display ==
  Data : Inport
  Bus Selector : BusSelector  OutputSignals=VirtualSensors.DrvInvtr.DrvMtrTrq [Nm]
  CmprTo : Blocks_lib/CmprTo  Commented=on  op===  val='Rev'  enum=EnumLst.PRNDMode
  Header : Blocks_lib/Header  width=Portrait  addtext=''
  RelOp(w/Hyst) : Blocks_lib/RelOp(w//Hyst)  relop=<
  raptor_adjustment : Raptor_lib/Data Storage/raptor_adjustment  paramName='DrvMtrTorq2RegenActive'  nameSource=Parameter  initValue=[-1 -5]  dataType=double  storage=Calibration  calDispType=Number  calEnum={'False', 'True'}  calGain=1.0  calOffset=0.0  calMax=inf  calMin=-inf  calFormat='-1'  calUnit='Nm'  calHelp='Values to display regen active, with hysteresis'  calAccess=1  calFunction='Control | Other'  calDispHeaders=off  calColHeaders={'Col1' 'Col2' 'Col3'}  calRowHeaders={'Row1' 'Row2' 'Row3'}
      settings: SourceProductName=Raptor
  Ctrl : Outport  VectorParamsAs1DForOutWhenUnconnected=off
  wires:
  RelOp(w/Hyst)/1 -> Ctrl/1  "Regenstate"
  Bus Selector/1 -> RelOp(w/Hyst)/1  "<DrvMtrTrq [Nm]>"
  Data/1 -> Bus Selector/1
  raptor_adjustment/1 -> RelOp(w/Hyst)/2

== system VCMGCM1962020b_v2/Fgnd/Control/Other/Other/FMWS ==
  note: This subsystem is for non-j1939 use
  Data : Inport
  Bus Selector : BusSelector  OutputSignals=Sensors.Sensors.Driver.Drv.Drv [Bool],Sensors.Sensors.Driver.Ntrl.Ntrl [Bool],Sensors.Sensors.Driver.Rev.Rev [Bool],VirtualSensors.Driver.Prk [Bool]
  Chart : Stateflow chart  Commented=on
  Chart1 : Stateflow chart
  Header : Blocks_lib/Header  width=Portrait  addtext=''
  Ctrl : Outport  VectorParamsAs1DForOutWhenUnconnected=off
  wires:
  Data/1 -> Bus Selector/1
  Bus Selector/1 -> Chart1/1(Drv)  "<Drv [Bool]>"
  Bus Selector/2 -> Chart1/2(Ntrl)  "<Ntrl [Bool]>"
  Bus Selector/3 -> Chart1/3(Rev)  "<Rev [Bool]>"
  Chart1/1(FMWS_State_gear) -> Ctrl/1  "FMWS_StateGear [enum]"
  Bus Selector/4 -> Chart1/4(Prk)  "<Prk [Bool]>"

== system VCMGCM1962020b_v2/Fgnd/Control/Other/Other/Lights & Lamps ==
  Data : Inport
  Bus Creator : BusCreator  Inputs=2
  Bus Selector : BusSelector  OutputSignals=VirtualSensors.Driver.BrkSw [Bool],Control.Mode.PRNDMode [enum]
  CmprTo : Blocks_lib/CmprTo  op===  val='Rev'  enum=EnumLst.PRNDMode
  Header : Blocks_lib/Header  width=Portrait  addtext=''
  Zero-Order Hold : ZeroOrderHold  SampleTime=-1
  Ctrl : Outport  VectorParamsAs1DForOutWhenUnconnected=off
  wires:
  Bus Creator/1 -> Ctrl/1  "Lamp"
  CmprTo/1 -> Bus Creator/2  "RevLight [Bool]"
  Zero-Order Hold/1 -> Bus Creator/1  "BrkLight [Bool]"
  Bus Selector/1 -> Zero-Order Hold/1  "<BrkSw [Bool]>"
  Data/1 -> Bus Selector/1
  Bus Selector/2 -> CmprTo/1  "<PRNDMode [enum]>"

== system VCMGCM1962020b_v2/Fgnd/Control/PDU/High-Voltage Discharge Contactor/HV Discharge/EvalDiag ==
  status : Inport
  f : TriggerPort  TriggerType=function-call  VariantControl=(inherit)
      settings: CopyFcn=Stateflow.SLINSF.SimulinkMan.removeBlockPreDeleteFcn  PreDeleteFcn=Stateflow.SLINSF.SimulinkMan.unsafePredeleteFcn
  Header : Blocks_lib/Header  width=Portrait  addtext=''
  raptor_fault_def : Raptor_lib/Faults/raptor_fault_def  faultName='HVDschgFault'  persist=off  sticky=off  emisRelated=off  singleTrip=off  clearMethod=Standard  xLimit=1  yLimit=1  calEnable=on  addDisable=off  calAccess=1  calFunction=['Diagnostics | Fault Defs | ' raptor_get_param_eval(gcb, 'faultName')]
      settings: SourceProductName=Raptor
  wires:
  status/1 -> raptor_fault_def/1

== system VCMGCM1962020b_v2/Fgnd/Control/PDU/Main  Contactor Cmd/Enable ==
  Data : Inport
  Bus Selector : BusSelector  OutputSignals=Control.Mode.StartStop.MainCntrReq [Bool]
  Header : Blocks_lib/Header  width=Portrait  addtext=''
  Logical Operator : Logic  Operator=NOT  Inputs=1  AllPortsSameDT=off  OutDataTypeStr=boolean
  Logical Operator1 : Logic  Inputs=3  AllPortsSameDT=off  OutDataTypeStr=boolean
  raptor_adjustment : Raptor_lib/Data Storage/raptor_adjustment  paramName=[nam 'PreChgEnbl']  nameSource=Parameter  initValue=0  dataType=boolean  storage=Calibration  calDispType=Number  calEnum={'False', 'True'}  calGain=1  calOffset=0  calMax=inf  calMin=-inf  calFormat=''  calUnit='Bool'  calHelp='Pre-charge enable'  calAccess=1  calFunction=group  calDispHeaders=off  calColHeaders={'Col1' 'Col2' 'Col3'}  calRowHeaders={'Row1' 'Row2' 'Row3'}
      settings: SourceProductName=Raptor
  raptor_fault_status : Raptor_lib/Faults/raptor_fault_status  faultSource=Parameter  faultName='EStop2'  notOccurred=off  suspected=off  active=off  occurred=off  failedThisDC=on  testCmpltThisDC=off  failing=off  pending=off  confirmed=off  mil=off  permanent=off  ready=off  prevConfirmed=off  failedSinceClear=off  failedLastDC=off  prevMil=off
      settings: SourceProductName=Raptor
  Bool : Outport  VectorParamsAs1DForOutWhenUnconnected=off
  wires:
  Bus Selector/1 -> Logical Operator1/2  "<MainCntrReq [Bool]>"
  raptor_adjustment/1 -> Logical Operator1/1
  Logical Operator1/1 -> Bool/1
  Data/1 -> Bus Selector/1
  Logical Operator/1 -> Logical Operator1/3
  raptor_fault_status/1 -> Logical Operator/1
